simulink model "SOC_NN"  (R2022b)
settings: Solver=FixedStepAuto  StartTime=0.0  StopTime=timeVector(end)  FixedStep=stepSize  MaxStep=60  RelTol=1e-3  AbsTol=1e-3
InitFcn:
  | load SOC_SLdata
values from neighbouring files (symbols this model uses):
  BatteryNN =     [SOC_SLdata.mat]
  Ts = 10    [SOC_SLdata.mat]
  X_MAX = [4.23207255751 5.99961 26.28963]    [SOC_SLdata.mat]
  X_MIN = [2.79645479834 -18.0971537397 -10.3047309401]    [SOC_SLdata.mat]
libraries: sharedTrackingLibrary x1, deeplib x1
settings Model: Creator=jgazzarr  LastModifiedBy=ppanares
settings SolverCC: AutoScaleAbsTol=off  AlgebraicLoopSolver=TrustRegion
settings OptimizationCC: DefaultParameterBehavior=Inlined  EnhancedBackFolding=on  PassReuseOutputArgsAs=Individual arguments  ZeroExternalMemoryAtStartup=off  ZeroInternalMemoryAtStartup=off  OptimizeBlockOrder=speed  DifferentSizesBufferReuse=on  OptimizationCustomize=off  EfficientTunableParamExpr=on
settings DebuggingCC: ParameterTunabilityLossMsg=error  UnconnectedInputMsg=warning  UnconnectedOutputMsg=warning  UnconnectedLineMsg=warning  SymbolicDimsDataTypeCodeGenerationDiagnostic=none  SFMachineParentedDataDiag=warning
settings HardwareCC: ProdBitPerPointer=32  ProdBitPerSizeT=32  ProdBitPerPtrDiffT=32  ProdWordSize=32  ProdHWDeviceType=Intel->x86-32 (Windows32)
settings ModelReferenceCC: EnableRefExpFcnMdlSchedulingChecks=on
settings SFSimCC: MATLABDynamicMemAlloc=off  CustomCodeUndefinedFunction=UseInterfaceOnly  SimTargetLang=C++
settings RTWCC: Description=Embedded Coder  SystemTargetFile=ert.tlc  TemplateMakefile=ert_default_tmf  GenerateReport=on  CustomInclude=C:\MATLAB\R2020b\extern\include\mkldnn  PortableWordSizes=on  CodeExecutionProfiling=on  CodeProfilingSaveOptions=MetricsOnly  CodeProfilingInstrumentation=detailed  GenerateCodeMetricsReport=on  DLArmComputeVersion=19.05  DLArmComputeArch=armv8
settings CodeAppCC: ForceParamTrailComments=on  IgnoreCustomStorageClasses=off  OperatorAnnotations=on  SimulinkDataObjDesc=on  SFDataObjDesc=on  InsertBlockDesc=on
settings ERTTargetCC: TargetLangStandard=C99 (ISO)  GenerateSampleERTMain=on  SupportContinuousTime=on  InlinedParameterPlacement=NonHierarchical  RootIOFormat=Structure reference  ERTCustomFileTemplate=example_file_process.tlc
settings SimscapeCC: SimscapeLogType=all  SimscapeLogSimulationStatistics=on  SimscapeLogDataHistory=10000

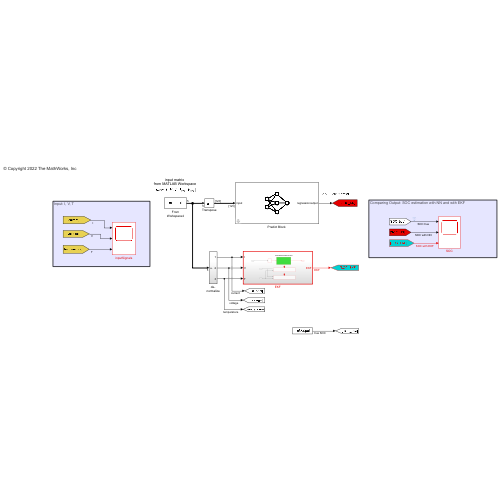
[thumbnail: Simulink's stored preview of the top-level diagram]
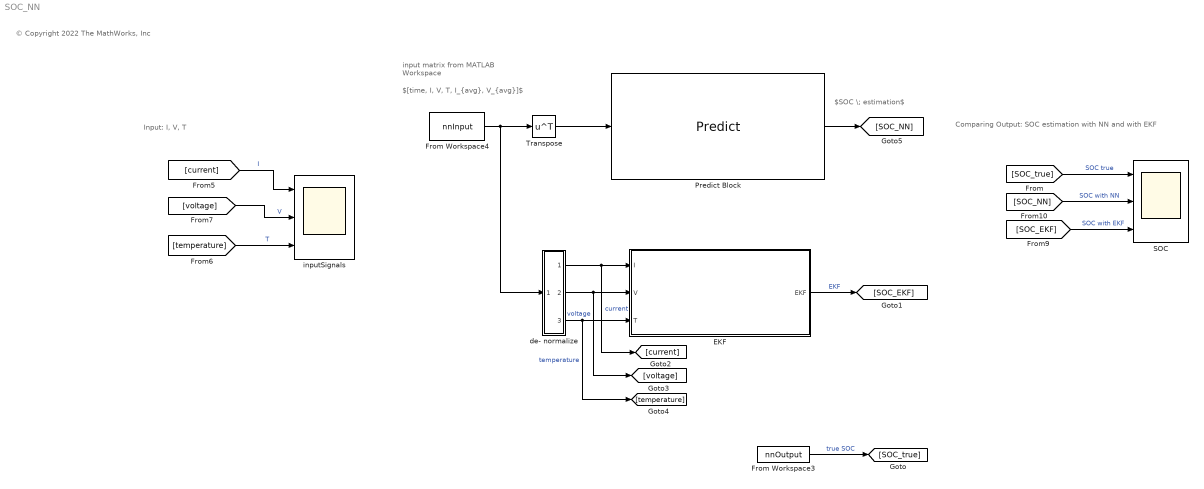
== system SOC_NN ==
  note: © Copyright 2022 The MathWorks, Inc
  note: Input: I, V, T
  note: Comparing Output: SOC estimation with NN and with EKF
  note: $SOC \; estimation$
  note: input matrix
      | from MATLAB Workspace
  note: $[time, I, V, T, I_{avg}, V_{avg}]$
  EKF : Subsystem  TreatAsAtomicUnit=on
  From Workspace3 : FromWorkspace  VariableName=nnOutput
  From Workspace4 : FromWorkspace  VariableName=nnInput
  "Predict Block " : deeplib/Predict  Network=Network from MAT-file  NetworkFunction=squeezenet  NetworkFilePath=net.mat  MiniBatchSize=128  InputDataFormats={ '', '' }  Predictions=on  Activations={}  ForceInterpretedSim=off  EnableDLNetwork=on
  SOC : Scope  NumInputPorts=3
  Transpose : Math  Operator=transpose
  de- normalize : Subsystem
  inputSignals : Scope  NumInputPorts=3
  wires:
  EKF/1(EKF) -> [SOC_EKF]  "EKF"
  de- normalize/1(Out1) -> [current], EKF/1(I)  "current"
  de- normalize/3(Out3) -> [temperature], EKF/3(T)  "temperature"
  de- normalize/2(Out2) -> [voltage], EKF/2(V)  "voltage"
  [current] -> inputSignals/1  "I"
  [voltage] -> inputSignals/2  "V"
  [temperature] -> inputSignals/3  "T"
  [SOC_true] -> SOC/1  "SOC true"
  [SOC_EKF] -> SOC/3  "SOC with EKF"
  [SOC_NN] -> SOC/2  "SOC with NN"
  Transpose/1 -> "Predict Block "/1
  "Predict Block "/1 -> [SOC_NN]
  From Workspace3/1 -> [SOC_true]  "true SOC"
  From Workspace4/1 -> de- normalize/1(u), Transpose/1

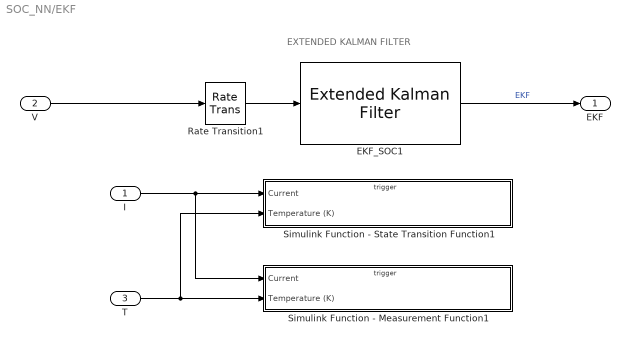
== system SOC_NN/EKF ==
  note: EXTENDED KALMAN FILTER
  I : Inport
  V : Inport  Port=2
  T : Inport  Port=3
  EKF_SOC1 : sharedTrackingLibrary/Extended Kalman Filter  StateTransitionFcn=batteryStateFcn  HasStateTransitionJacobianFcn=off  HasAdditiveProcessNoise=Additive  ProcessNoise=1e-4  HasTimeVaryingProcessNoise=off  HasStateTransitionFcnExtraArgument=0  InitialState=1  InitialStateCovariance=1e-2  MeasurementFcn1=batteryMeasurementFcn  HasMeasurementJacobianFcn1=off  HasMeasurementEnablePort1=off  HasAdditiveMeasurementNoise1=Additive  MeasurementNoise1=0.5  HasTimeVaryingMeasurementNoise1=off  HasMeasurementFcnExtraArgument1=0  HasMeasurementWrapping1=off  MeasurementFcn2=myMeasurementFcn  HasMeasurementJacobianFcn2=off  HasMeasurementEnablePort2=off  HasAdditiveMeasurementNoise2=Additive  MeasurementNoise2=1  HasTimeVaryingMeasurementNoise2=off  HasMeasurementFcnExtraArgument2=0  HasMeasurementWrapping2=off  MeasurementFcn3=myMeasurementFcn  HasMeasurementJacobianFcn3=off  HasMeasurementEnablePort3=off  HasAdditiveMeasurementNoise3=Additive  MeasurementNoise3=1  HasTimeVaryingMeasurementNoise3=off  HasMeasurementFcnExtraArgument3=0  HasMeasurementWrapping3=off  MeasurementFcn4=myMeasurementFcn  HasMeasurementJacobianFcn4=off  HasMeasurementEnablePort4=off  HasAdditiveMeasurementNoise4=Additive  MeasurementNoise4=1  HasTimeVaryingMeasurementNoise4=off  HasMeasurementFcnExtraArgument4=0  HasMeasurementWrapping4=off  MeasurementFcn5=myMeasurementFcn  HasMeasurementJacobianFcn5=off  HasMeasurementEnablePort5=off  HasAdditiveMeasurementNoise5=Additive  MeasurementNoise5=1  HasTimeVaryingMeasurementNoise5=off  HasMeasurementFcnExtraArgument5=0  HasMeasurementWrapping5=off  EnableMultirate=off  StateTransitionFcnSampleTime=1  MeasurementFcn1SampleTime=1  MeasurementFcn2SampleTime=1  MeasurementFcn3SampleTime=1  MeasurementFcn4SampleTime=1  MeasurementFcn5SampleTime=1  UseCurrentEstimator=on  OutputStateCovariance=off  DataType=double  SampleTime=Ts  NumberOfMeasurements=1
  Rate Transition1 : RateTransition
  Simulink Function - Measurement Function1 : Subsystem  TreatAsAtomicUnit=on
  Simulink Function - State Transition Function1 : Subsystem  TreatAsAtomicUnit=on
  EKF : Outport  VectorParamsAs1DForOutWhenUnconnected=off
  wires:
  I/1 -> Simulink Function - Measurement Function1/1(Current), Simulink Function - State Transition Function1/1(Current)
  T/1 -> Simulink Function - State Transition Function1/2(Temperature (K)), Simulink Function - Measurement Function1/2(Temperature (K))
  V/1 -> Rate Transition1/1
  Rate Transition1/1 -> EKF_SOC1/1
  EKF_SOC1/1 -> EKF/1  "EKF"

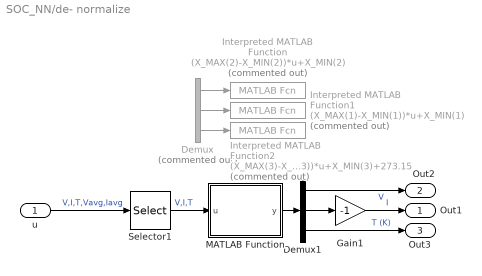
== system SOC_NN/de- normalize ==
  u : Inport
  Demux : Demux  Commented=on  Outputs=3
  Demux1 : Demux  Outputs=3
  Gain1 : Gain  Gain=-1
  Interpreted MATLAB Function : MATLABFcn  Commented=on  MATLABFcn=(X_MAX(2)-X_MIN(2))*u+X_MIN(2)
  Interpreted MATLAB Function1 : MATLABFcn  Commented=on  MATLABFcn=(X_MAX(1)-X_MIN(1))*u+X_MIN(1)
  Interpreted MATLAB Function2 : MATLABFcn  Commented=on  MATLABFcn=(X_MAX(3)-X_MIN(3))*u+X_MIN(3)+273.15
  MATLAB Function : MATLAB Function  TreatAsAtomicUnit=on
  Selector1 : Selector  InputPortWidth=5  IndexOptions=Index vector (dialog)  Indices=[1 2 3]  OutputSizes=1
  Out1 : Outport
  Out2 : Outport  Port=2
  Out3 : Outport  Port=3
  wires:
  Demux/3 -> Interpreted MATLAB Function2/1
  Demux/1 -> Interpreted MATLAB Function/1
  u/1 -> Selector1/1  "V,I,T,Vavg,Iavg"
  Demux/2 -> Interpreted MATLAB Function1/1
  MATLAB Function/1(y) -> Demux1/1
  Demux1/3 -> Out3/1  "T (K)"
  Demux1/1 -> Out2/1  "V"
  Demux1/2 -> Gain1/1
  Selector1/1 -> MATLAB Function/1(u)  "V,I,T"
  Gain1/1 -> Out1/1  "I"

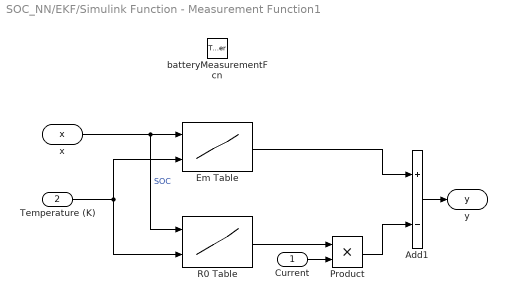
== system SOC_NN/EKF/Simulink Function - Measurement Function1 ==
  Current : Inport
  Temperature (K) : Inport  Port=2
  batteryMeasurementFcn : TriggerPort  TriggerType=function-call  IsSimulinkFunction=on  FunctionName=batteryMeasurementFcn  FunctionVisibility=scoped  VariantControl=Variant
  Add1 : Sum  Inputs=+-
  Em Table : Lookup_n-D  BreakpointsForDimension1=BatteryNN.SOC_LUT  BreakpointsForDimension2=BatteryNN.Temperature_LUT  Table=BatteryNN.Em_LUT  InternalRulePriority=Speed  RndMeth=Simplest
      settings: InputPortMap=u0,u1
  Product : Product
  R0 Table : Lookup_n-D  BreakpointsForDimension1=BatteryNN.SOC_LUT  BreakpointsForDimension2=BatteryNN.Temperature_LUT  Table=BatteryNN.R0_LUT  InternalRulePriority=Speed  RndMeth=Simplest
      settings: InputPortMap=u0,u1
  x : ArgIn  DisableCoverage=on  ArgumentName=x
  y : ArgOut  DisableCoverage=on  ArgumentName=y
  wires:
  x/1 -> R0 Table/1, Em Table/1  "SOC"
  Em Table/1 -> Add1/1
  Add1/1 -> y/1
  Temperature (K)/1 -> R0 Table/2, Em Table/2
  R0 Table/1 -> Product/1
  Current/1 -> Product/2
  Product/1 -> Add1/2

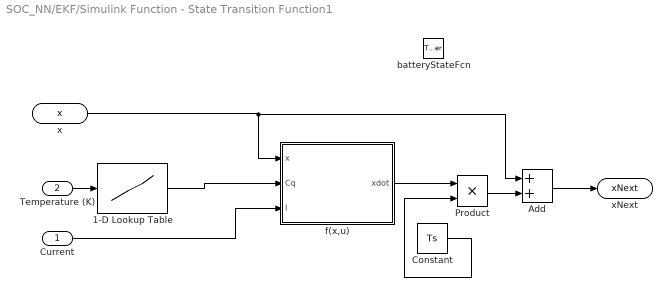
== system SOC_NN/EKF/Simulink Function - State Transition Function1 ==
  Current : Inport
  Temperature (K) : Inport  Port=2
  batteryStateFcn : TriggerPort  TriggerType=function-call  IsSimulinkFunction=on  FunctionName=batteryStateFcn  FunctionVisibility=scoped  VariantControl=Variant
  1-D Lookup Table : Lookup_n-D  NumberOfTableDimensions=1  BreakpointsForDimension1=BatteryNN.Temperature_LUT  Table=BatteryNN.Capacity_LUT  InternalRulePriority=Speed  RndMeth=Simplest
  Add : Sum
  Constant : Constant  Value=Ts  OutDataTypeStr=single
  Product : Product  OutDataTypeStr=single
  f(x,u) : MATLAB Function  TreatAsAtomicUnit=on
  x : ArgIn  DisableCoverage=on  ArgumentName=x
  xNext : ArgOut  DisableCoverage=on  ArgumentName=xNext
  wires:
  x/1 -> f(x,u)/1(x), Add/1
  Add/1 -> xNext/1
  Constant/1 -> Product/2
  f(x,u)/1(xdot) -> Product/1
  Product/1 -> Add/2
  Current/1 -> f(x,u)/3(I)
  1-D Lookup Table/1 -> f(x,u)/2(Cq)
  Temperature (K)/1 -> 1-D Lookup Table/1

== matlab function SOC_NN/de- normalize/MATLAB Function ==
  data: u input; y output; X_MAX parameter; X_MIN parameter
function y = fcn(u, X_MAX, X_MIN)
y = (X_MAX-X_MIN).*u+X_MIN;
y(3) = y(3) + 273.15; % convert to K

== matlab function SOC_NN/EKF/Simulink Function - State Transition Function1/f(x,u) ==
  data: x input; Cq input; I input; xdot output
function xdot = fx(x,Cq,I)
% function xdot = fx(x,R1,R2,R3,t1,t2,t3,Cq,I)
xdot = zeros(size(x));
% U1 = x(2);
% U2 = x(3);
% U3 = x(4);
xdot(1) = -I/(3600*Cq);
% xdot(2) = -1/t1*U1 + I/(t1/R1);
% xdot(3) = -1/t2*U2 + I/(t2/R2);
% xdot(4) = -1/t3*U3 + I/(t3/R3);
